simulink model "Simplified_LVDCMG4PQ"  (R2017a)
settings: Solver=FixedStepDiscrete  StartTime=0.0  StopTime=SimStopTime  FixedStep=Td  RelTol=1e-3  EnableMultiTasking=on
PostLoadFcn:
  | , if any(exist('dsrtsu_mdlpostloadfcn', 'file') == [2, 3, 6]), try dsrtsu_mdlpostloadfcn('Execute', bdroot); catch fprintf('Error in PostLoadFcn (dsrtsu_mdlpostloadfcn) for model "%s":\n %s\n', bdroot, lasterr); end, end,
InitFcn:
  | clc;
  | clear all;
  | % ----sampling time---------
  | SimStopTime=2;
  | Tch = inf;
  | Td = 1/500000 % 1/fs = sampling period
  | Fd=1/Td
  | Ts = Td;
  | T_simplified_simul=1/10000;
  | T_pq_ctr=1/10000;
  | Fpwm=10000;
  | 
  | Vsource=400;% not sure it is used - !!!! - pls check
  | 
  | %------DC to DC boost Converter-------------
  | stepTimeSource=SimStopTime-1.5;
  | fGrid=50; %Hz grid frequency
  | HarmonicOrd=6;%comming from inverter/grid
  | Vin=24; %volts
  | L_boost=0.5e-3;
  | C_boost=50e-6;
  | stepTimeDutyCl=stepTimeSource+0.01;
  | stepTime1Load= stepTimeSource-0.3; %11.5;
  | stepTime2Load=SimStopTime-0.5; %19
  | 
  | % parameters for AC/DC inverter - not used here
  | %Kp_cc=23.5;
  | %Ki_cc=909;
  | %Ti_cc=1/909;
  | %Ki_har=1000;
  | %Ki_neg=4000;
  | Tsampling=T_pq_ctr;
  | Tdelay=1.5*T_pq_ctr; %not sure it is used anywhere
  | 
  | %R_gsc_on=0.001;
  | 
  | %V_dc_link_initial=735;
  | %C_dc_link=1100e-6;
  | %C_dc_link=1100e-6;
  | 
  | %Inomin=10.25; %for Sinv_rating=5kVA
  | %Vnomin=325;
  | 
  | %Tsampling=-1;
  | %Fil_nom=0.011;
  | %Fil_dom=0.989;
  | %Fil_nom_he=0.075;
  | %Fil_dom_he=0.925;
  | %wf=(2*pi*50)/sqrt(2);
  | %NOM=(wf*T_pq_ctr)/(1+wf*T_pq_ctr)
  | %DOM=1/(1+wf*T_pq_ctr)
  | %Fil_nom=NOM;
  | %Fil_dom=DOM;
  | %Fil_nom_he=NOM;
  | %Fil_dom_he=DOM;
  | 
  | %wf=(2*pi*1);
  | %NOMf=(wf*T_pq_ctr)/(1+wf*T_pq_ctr)
  | %DOMf=1/(1+wf*T_pq_ctr)
  | 
  | 
  | %FVabc_nom=0.5;
  | %FVabc_dom=0.5;
  | 
  | 
  | %PLL
  | %Tset = 0.1    % settling time
  | %zeta = 0.7   % damping ratio (optimized for best response of the second order TF
  | 
  | % initialisation of current controller
  | %oc = 2*pi*50
  | %R_grid=2;
  | %L_grid=5/1000;
  | %R_grid=0.2;
  | %L_grid=4/1000;
  | %Ltranf=1/1000;
  | %C_filter=4.7/1000000;
  | 
  | %R_conv1=0.5;
  | %L_conv1=24/1000;
  | %R_conv2=0.5;
  | %L_conv2=1.5/1000;
  | %C_f=1/1000000;
  | %R_f=12.57;
  | 
  | %parameters
  | %R_conv=0.5; % 0.1 Ohm
  | %L_conv=15.8/1000; %1.8 mH
  | %R_conv=R_conv1+R_conv2;
  | %L_conv=L_conv1+L_conv2;
  | %R_tot=R_conv1+R_conv2;
  | %L_tot=L_conv1+L_conv2;
  | %T_tot=L_tot/R_tot;
  | 
  | %FDIA
  | %n_pi=0.008;
  | %n_pd=0.01;
  | %DELTA_ALPHA=(1.1/0.9-1)*(R_conv*T_pq_ctr)/L_conv;
  | %DELTA_BETA=(1/0.9-1)*(T_pq_ctr/L_conv);
  | 
  | 
  | %UdcTransdRatio = 25e-3/800
  | %UaTransdRatio = 25e-3/600
  | %UbTransdRatio = 25e-3/600
  | %UcTransdRatio = 25e-3/600
  | 
  | 
  | %RMeasIa = 220;
  | %RMeasIb = 220;
  | %RMeasIc = 220;
  | %RMeasIdc = 220;
  | %RMeasUd = 220;
  | %RMeasUa = 220;
  | %RMeasUb = 220;
  | %RMeasUc = 220;
  | 
  | %LemTurnsIa = 5
  | %LemTurnsIb = 5;
  | %LemTurnsIc = 5;
  | %LemTurnsIdc = 5;
  | 
  | %IaTransdRatio = LemTurnsIa/1000
  | %IbTransdRatio = LemTurnsIb/1000
  | %IcTransdRatio = LemTurnsIc/1000
  | %IdcTransdRatio = LemTurnsIdc/1000
undefined symbols (not defined in the file): C_dc_link, V_dc_link_initial
libraries: powerlib x22, simulink x1
settings Model: DSRTSU_INTERNAL_RTI_VER=380  DSRTSU_INTERNAL_RTI_TYPE=rti1103  Creator=peres  LastModifiedBy=me
settings DataIOCC: LimitDataPoints=on  SaveFormat=Array  SignalLoggingSaveFormat=ModelDataLogs
settings OptimizationCC: BlockReduction=off  ConditionallyExecuteInputs=off  OptimizeBlockIOStorage=off  BufferReuse=off  GlobalBufferReuse=off  ExpressionFolding=off  ExpressionDepthLimit=2147483647  LocalBlockOutputs=off  InitFltsAndDblsToZero=on  LifeSpan=inf
settings DebuggingCC: SaveWithParameterizedLinksMsg=none  UnderspecifiedInitializationDetection=Classic  MergeDetectMultiDrivingBlocksExec=none  SignalResolutionControl=TryResolveAllWithWarning  SolverPrmCheckMsg=warning  MultiTaskDSMMsg=warning  MultiTaskCondExecSysMsg=none  FcnCallInpInsideContextMsg=warning  AllowSymbolicDim=off  StateNameClashWarn=warning  SFUnexpectedBacktrackingDiag=warning  SFNoUnconditionalDefaultTransitionDiag=warning  SFExecutionAtInitializationDiag=none
settings HardwareCC: ProdBitPerPointer=32  ProdBitPerSizeT=32  ProdBitPerPtrDiffT=32  ProdLargestAtomicFloat=None  ProdEndianess=BigEndian  ProdWordSize=32  ProdHWDeviceType=Generic->Custom  TargetIntDivRoundTo=Zero  TargetEndianess=BigEndian  TargetHWDeviceType=Generic->Custom
settings ModelReferenceCC: PropagateSignalLabelsOutOfModel=off
settings RTWCC: SystemTargetFile=rti1103.tlc  MakeCommand=make_rti  TemplateMakefile=rti1103.tmf  Description=dSPACE DS1103 Hardware Platform  RTWVerbose=off
settings STFCustomTargetCC: TargetFcnLib=ansi_tfl_tmw.mat  ParMdlRefBuildCompliant=on  GeneratePreprocessorConditionals=Disable all  CPPClassGenCompliant=on  SystemTargetFile=rti1103.tlc
settings GRTTargetCC: TargetFcnLib=ansi_tfl_tmw.mat  TargetLangStandard=C89/C90 (ANSI)  CompOptLevelCompliant=off  ConcurrentExecutionCompliant=off  GeneratePreprocessorConditionals=Disable all  CombineOutputUpdateFcns=off  MatFileLogging=off  GRTInterface=on  UseToolchainInfoCompliant=off  ExtModeMexFile=noextcomm
settings ConfigComp: CovMetricSettings=dw  CovHtmlReporting=on  CovSaveCumulativeToWorkspaceVar=on  CovSaveSingleToWorkspaceVar=on  CovExternalEMLEnable=off

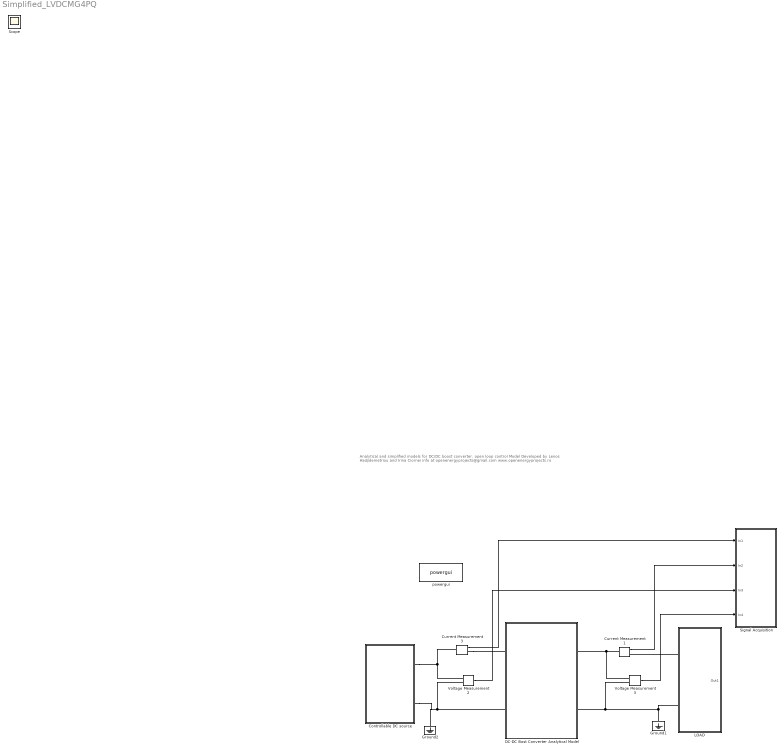
== system Simplified_LVDCMG4PQ ==
  note: Analytical and simplified models for DC/DC boost converter, open loop control
      |
      | Model Developed by Lenos Hadjidemetriou and Irina Ciornei
      | info at openenergyprojects@gmail.com
      | www.openenergyprojects.ro
  Controllable DC source : Subsystem
  Current Measurement1 : powerlib/Measurements/Current Measurement  PhasorSimulation=off  OutputType=Complex  PSBequivalent=0
  Current Measurement3 : powerlib/Measurements/Current Measurement  PhasorSimulation=off  OutputType=Complex  PSBequivalent=0
  DC-DC Bost Converter Analytical Model : Subsystem
  Ground1 : powerlib/Elements/Ground  LConnTagsString=a
  Ground2 : powerlib/Elements/Ground  LConnTagsString=a
  LOAD : Subsystem
  Signal Acquisition : Subsystem
  Voltage Measurement2 : powerlib/Measurements/Voltage Measurement  PhasorSimulation=off  OutputType=Complex  PSBequivalent=0
  Voltage Measurement3 : powerlib/Measurements/Voltage Measurement  PhasorSimulation=off  OutputType=Complex  PSBequivalent=0
  powergui : powerlib/powergui  Priority=1  SimulationMode=Discrete  SampleTime=Td  frequency=60  Iterations=50  frequencyindice=0  Pbase=100e6  ErrMax=1e-4  UnitsV=kV  UnitsW=MW  buscounter=0  FunctionMessages=off  echomessages=off  EnableUseOfTLC=off  CurrentSourceSwitches=off  DisableSnubberDevices=off  DisableRonSwitches=off  DisableVfSwitches=off  DisplayEquations=off  SolverType=Tustin  Interpol=off  ExternalGateDelay=off  methode=off  Ts=0  x0status=blocks  SPID=off  SwTol=0  HookPort=off  RestoreLinks=warning  ResistiveCurrentMeasurement=off  Frange=[0:2:500]  Ylog=off  Xlog=on  ShowGrid=off  save=off  variable=ZData  structure=Vref  ZoomFFT=on  StartTime=0.66  cycles=1  DisplayStyle=1  fundamental=50  FreqAxis=on  MaxFrequency=2000  frequencyindicesteady=1  RmsSteady=1  display=off
  Scope : Scope
  wires:
  Current Measurement3/1 -> Signal Acquisition/1(In1)
  Current Measurement1/1 -> Signal Acquisition/2(In2)
  Voltage Measurement2/1 -> Signal Acquisition/3(In3)
  Voltage Measurement3/1 -> Signal Acquisition/4(In4)
  connections:
  Voltage Measurement3/LConn2 -- DC-DC Bost Converter Analytical Model/RConn2 -- LOAD/LConn2 -- Ground1/LConn1
  Voltage Measurement2/LConn2 -- DC-DC Bost Converter Analytical Model/LConn2 -- Ground2/LConn1 -- Controllable DC source/RConn2
  Voltage Measurement2/LConn1 -- Current Measurement3/LConn1 -- Controllable DC source/RConn1
  Current Measurement3/RConn1 -- DC-DC Bost Converter Analytical Model/LConn1
  Current Measurement1/LConn1 -- DC-DC Bost Converter Analytical Model/RConn1 -- Voltage Measurement3/LConn1
  LOAD/LConn1 -- Current Measurement1/RConn1

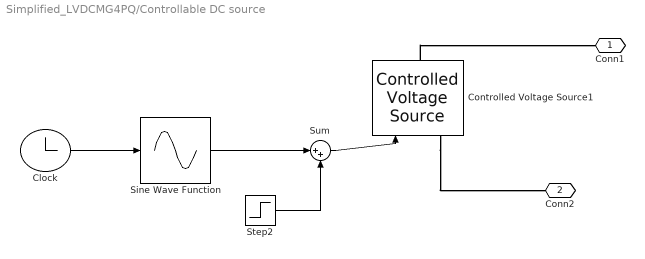
== system Simplified_LVDCMG4PQ/Controllable DC source ==
  Clock : Clock
  Controlled Voltage Source1 : powerlib/Electrical Sources/Controlled Voltage Source  Initialize=on  Source_Type=DC  Amplitude=Vin  Phase=0  Frequency=0  Measurements=None
  Sine Wave Function : Sin  TimeSource=Use external signal  Amplitude=0.3/Vin  Bias=Vin  Frequency=2*pi*fGrid*HarmonicOrd  SampleTime=0
  Step2 : Step  Time=stepTimeSource
  Sum : Sum  Inputs=|++
  Conn1 : PMIOPort  Port=1  Side=Right
  Conn2 : PMIOPort  Port=2  Side=Right
  wires:
  Sine Wave Function/1 -> Sum/1
  Clock/1 -> Sine Wave Function/1
  Step2/1 -> Sum/2
  Sum/1 -> Controlled Voltage Source1/1
  connections:
  Controlled Voltage Source1/LConn1 -- Conn2/RConn1
  Controlled Voltage Source1/RConn1 -- Conn1/RConn1

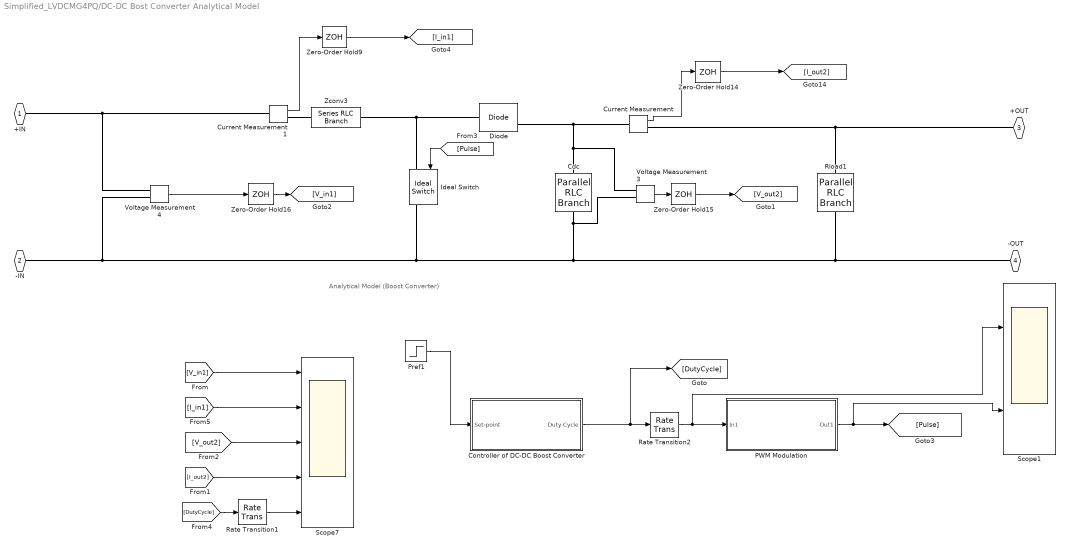
== system Simplified_LVDCMG4PQ/DC-DC Bost Converter Analytical Model ==
  note: Analytical Model (Boost Converter)
  Cdc : powerlib/Elements/Parallel RLC Branch  LConnTagsString=a  RConnTagsString=__new0  BranchType=C  Resistance=1  Inductance=1e-3  SetiL0=off  InitialCurrent=0  Capacitance=C_boost  Setx0=on  InitialVoltage=0  Measurements=None
  Controller of DC-DC Boost Converter : Subsystem
  Current Measurement : powerlib/Measurements/Current Measurement  PhasorSimulation=off  OutputType=Complex  PSBequivalent=0
  Current Measurement1 : powerlib/Measurements/Current Measurement  PhasorSimulation=off  OutputType=Complex  PSBequivalent=0
  Diode : powerlib/Power Electronics/Diode  Ron=0.0000001  Lon=0  Vf=0.0000001  IC=0  UseSnubber=off  Rs=5000000000  Cs=250e-6  Measurements=on
  Ideal Switch : powerlib/Power Electronics/Ideal Switch  Ron=0.00000001  Lon=0  IC=0  Rs=1e12  Cs=inf  Measurements=on
  PWM Modulation : Subsystem
  Pref1 : Step  Time=stepTimeDutyCl  Before=0.4  After=0.48  SampleTime=Tsampling
  Rate Transition1 : RateTransition
  Rate Transition2 : RateTransition  OutPortSampleTime=Td
  Rload1 : powerlib/Elements/Parallel RLC Branch  LConnTagsString=a  RConnTagsString=__new0  BranchType=R  Resistance=10000  Inductance=1e-3  SetiL0=off  InitialCurrent=0  Capacitance=C_dc_link*2  Setx0=on  InitialVoltage=V_dc_link_initial/2  Measurements=None
  Scope1 : Scope  NumInputPorts=2
  Scope7 : Scope  NumInputPorts=5
  Voltage Measurement3 : powerlib/Measurements/Voltage Measurement  PhasorSimulation=off  OutputType=Complex  PSBequivalent=0
  Voltage Measurement4 : powerlib/Measurements/Voltage Measurement  PhasorSimulation=off  OutputType=Complex  PSBequivalent=0
  Zconv3 : powerlib/Elements/Series RLC Branch  LConnTagsString=__new0  RConnTagsString=__new0  BranchType=L  Resistance=0.00001  Inductance=L_boost  SetiL0=off  InitialCurrent=0  Capacitance=1e-6  Setx0=off  InitialVoltage=0  Measurements=None
  Zero-Order Hold{9,14..16} (4 alike) : ZeroOrderHold  SampleTime=T_simplified_simul
  +IN : PMIOPort  Port=1  Side=Left
  -IN : PMIOPort  Port=2  Side=Left
  +OUT : PMIOPort  Port=3  Side=Right
  -OUT : PMIOPort  Port=4  Side=Right
  wires:
  Pref1/1 -> Controller of DC-DC Boost Converter/1(Set-point)
  Rate Transition1/1 -> Scope7/5
  [I_out2] -> Scope7/4
  PWM Modulation/1(Out1) -> [Pulse], Scope1/2
  Controller of DC-DC Boost Converter/1(Duty Cycle) -> [DutyCycle], Rate Transition2/1
  [DutyCycle] -> Rate Transition1/1
  [I_in1] -> Scope7/2
  [V_out2] -> Scope7/3
  Rate Transition2/1 -> PWM Modulation/1(In1), Scope1/1
  [V_in1] -> Scope7/1
  Zero-Order Hold15/1 -> [V_out2]
  Voltage Measurement3/1 -> Zero-Order Hold15/1
  [Pulse] -> Ideal Switch/1
  Zero-Order Hold9/1 -> [I_in1]
  Current Measurement/1 -> Zero-Order Hold14/1
  Voltage Measurement4/1 -> Zero-Order Hold16/1
  Zero-Order Hold16/1 -> [V_in1]
  Zero-Order Hold14/1 -> [I_out2]
  Current Measurement1/1 -> Zero-Order Hold9/1
  connections:
  -IN/RConn1 -- Ideal Switch/RConn1 -- Cdc/RConn1 -- Voltage Measurement3/LConn2 -- -OUT/RConn1 -- Rload1/RConn1 -- Voltage Measurement4/LConn2
  Voltage Measurement4/LConn1 -- +IN/RConn1 -- Current Measurement1/LConn1
  Current Measurement1/RConn1 -- Zconv3/RConn1
  +OUT/RConn1 -- Rload1/LConn1 -- Current Measurement/RConn1
  Current Measurement/LConn1 -- Diode/RConn1 -- Voltage Measurement3/LConn1 -- Cdc/LConn1
  Diode/LConn1 -- Zconv3/LConn1 -- Ideal Switch/LConn1

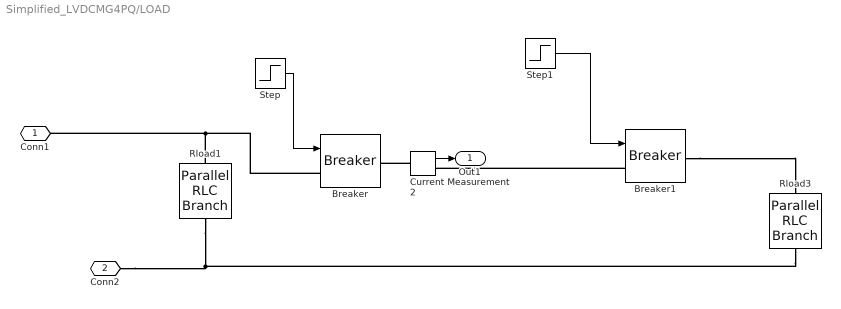
== system Simplified_LVDCMG4PQ/LOAD ==
  Breaker : powerlib/Elements/Breaker  InitialState=0  SwitchingTimes=[0.05 ]  External=on  BreakerResistance=0.01  SnubberResistance=1e6  SnubberCapacitance=inf  Measurements=None  MoreParameters=on  NoBreakLoop=off
      settings: SourceProductName=Simscape Power Systems
  Breaker1 : powerlib/Elements/Breaker  InitialState=1  SwitchingTimes=[0.05 ]  External=on  BreakerResistance=0.01  SnubberResistance=1e6  SnubberCapacitance=inf  Measurements=None  MoreParameters=on  NoBreakLoop=off
      settings: SourceProductName=Simscape Power Systems
  Current Measurement2 : powerlib/Measurements/Current Measurement  PhasorSimulation=off  OutputType=Complex  PSBequivalent=0
  Rload1 : powerlib/Elements/Parallel RLC Branch  LConnTagsString=a  RConnTagsString=__new0  BranchType=R  Resistance=114  Inductance=1e-3  SetiL0=off  InitialCurrent=0  Capacitance=C_dc_link*2  Setx0=on  InitialVoltage=V_dc_link_initial/2  Measurements=None
  Rload3 : powerlib/Elements/Parallel RLC Branch  LConnTagsString=a  RConnTagsString=__new0  BranchType=R  Resistance=114  Inductance=1e-3  SetiL0=off  InitialCurrent=0  Capacitance=C_dc_link*2  Setx0=on  InitialVoltage=V_dc_link_initial/2  Measurements=None
  Step : Step  Time=stepTime1Load  SampleTime=Td
  Step1 : Step  Time=stepTime2Load  Before=1  After=0  SampleTime=Td
  Conn1 : PMIOPort  Port=1  Side=Left
  Conn2 : PMIOPort  Port=2  Side=Left
  Out1 : Outport
  wires:
  Step/1 -> Breaker/1
  Step1/1 -> Breaker1/1
  Current Measurement2/1 -> Out1/1
  connections:
  Breaker/LConn1 -- Conn1/RConn1 -- Rload1/LConn1
  Breaker1/RConn1 -- Rload3/LConn1
  Breaker1/LConn1 -- Current Measurement2/RConn1
  Current Measurement2/LConn1 -- Breaker/RConn1
  Rload3/RConn1 -- Conn2/RConn1 -- Rload1/RConn1

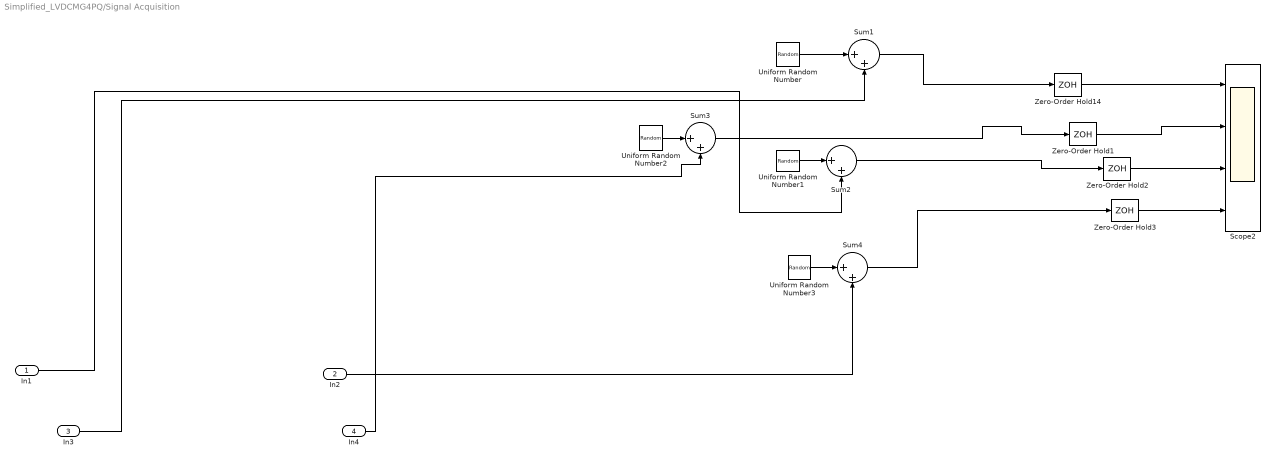
== system Simplified_LVDCMG4PQ/Signal Acquisition ==
  In1 : Inport
  In2 : Inport  Port=2
  In3 : Inport  Port=3
  In4 : Inport  Port=4
  Scope2 : Scope  NumInputPorts=4
  Sum{1..4} (4 alike) : Sum  Inputs=|++
  Uniform Random Number : UniformRandomNumber  Minimum=-0.001*Vin  Maximum=+0.001*Vin  Seed=1
  Uniform Random Number1 : UniformRandomNumber  Minimum=-0.005  Maximum=+0.005  Seed=1
  Uniform Random Number2 : UniformRandomNumber  Minimum=-0.001*48  Maximum=+0.001*48  Seed=1
  Uniform Random Number3 : UniformRandomNumber  Minimum=-0.5  Maximum=+0.5  Seed=1
  Zero-Order Hold{1..3,14} (4 alike) : ZeroOrderHold  SampleTime=T_simplified_simul
  wires:
  In1/1 -> Sum2/2
  In2/1 -> Sum4/2
  Uniform Random Number1/1 -> Sum2/1
  Sum3/1 -> Zero-Order Hold1/1
  Zero-Order Hold14/1 -> Scope2/1
  Sum1/1 -> Zero-Order Hold14/1
  In4/1 -> Sum3/2
  Uniform Random Number/1 -> Sum1/1
  In3/1 -> Sum1/2
  Sum4/1 -> Zero-Order Hold3/1
  Zero-Order Hold1/1 -> Scope2/2
  Zero-Order Hold3/1 -> Scope2/4
  Sum2/1 -> Zero-Order Hold2/1
  Uniform Random Number2/1 -> Sum3/1
  Zero-Order Hold2/1 -> Scope2/3
  Uniform Random Number3/1 -> Sum4/1

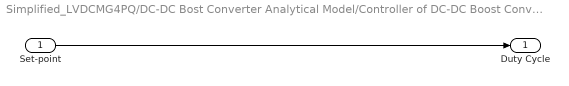
== system Simplified_LVDCMG4PQ/DC-DC Bost Converter Analytical Model/Controller of DC-DC Boost Converter ==
  Set-point : Inport
  Duty Cycle : Outport
  wires:
  Set-point/1 -> Duty Cycle/1

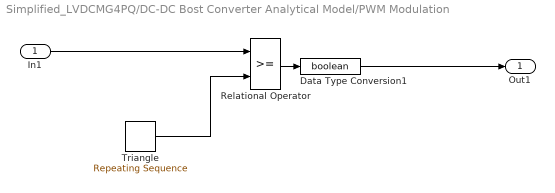
== system Simplified_LVDCMG4PQ/DC-DC Bost Converter Analytical Model/PWM Modulation ==
  In1 : Inport
  Data Type Conversion1 : DataTypeConversion  OutDataTypeStr=boolean  SampleTime=Ts  SaturateOnIntegerOverflow=on  RndMeth=Zero
  Relational Operator : RelationalOperator  SampleTime=Td  RndMeth=Nearest  InputSameDT=on
  Triangle : simulink/Sources/Repeating Sequence  rep_seq_t=[0 1/Fpwm/4 3/Fpwm/4 1/Fpwm]  rep_seq_y=[0.5 0 1 0.5]
  Out1 : Outport
  wires:
  In1/1 -> Relational Operator/1
  Data Type Conversion1/1 -> Out1/1
  Relational Operator/1 -> Data Type Conversion1/1
  Triangle/1 -> Relational Operator/2
